simulink model "Global_control_with_arbitraty_rate_of_convergence"  (R2021a)
settings: Solver=FixedStepDiscrete  StartTime=0.0  StopTime=12  FixedStep=1.0E-5  RelTol=1e-3
undefined symbols (not defined in the file): DiscIntNeverNeededParam, sigbuilder_block
libraries: simulink x4
(part 1 of 2)
settings Model: Creator=Mehra  LastModifiedBy=Mehra

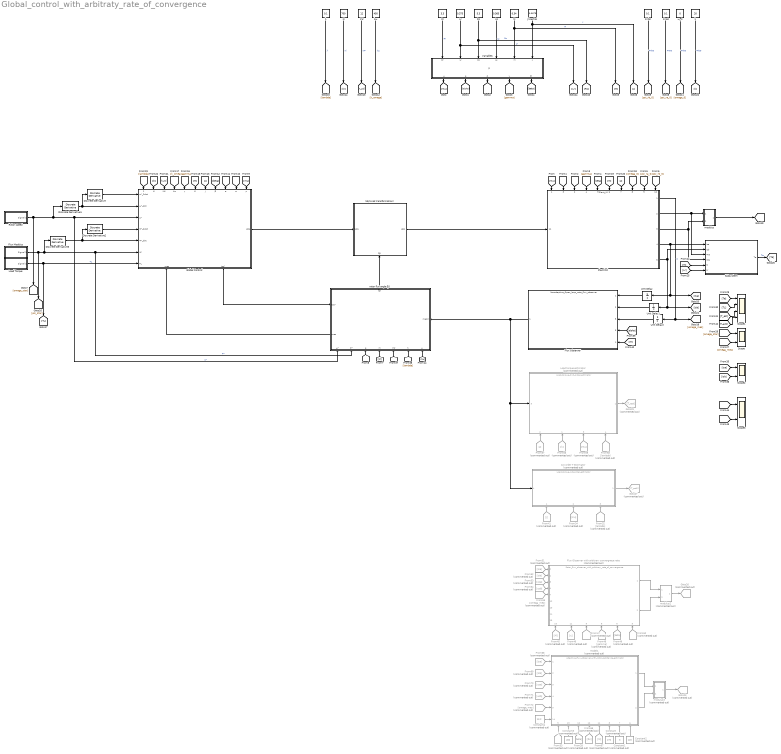
== system Global_control_with_arbitraty_rate_of_convergence ==
  note: β
  (dq to ab transformation) : Subsystem
      settings: PortSchema="{\"entries\":[{\"content\":{\"sides\":[{\"content\":{\"connectorIds\":[\"In1\"]},\"type\":\"ConnectorPlacement.EquallySpacedRectSide\",\"uuid\":\"fcc9e9c0-f3ff-45b3-b4d9-89988d9b9a34\"},{\"content\":{\"connectorIds\":[\"Out1\"],\"side\":\"RIGHT\"},\"type\":\"ConnectorPlacement.EquallySpacedRectSide\",\"uuid\":\"b8117d1c-eda8-48ca-a376-b80f3451eb1b\"},{\"content\":{\"connectorIds\":[],\"side\":\"TOP\"},\"type\":\"ConnectorPlacement.EquallySpacedRectSide\",\"uuid\":\"632a2e27-4ebf-4489-a7a1-4102ed33f7de\"},{\"content\":{\"connectorIds\":[\"In2\"],\"side\":\"BOTTOM\"},\"type\":\"ConnectorPlacement.EquallySpacedRectSide\",\"uuid\":\"b1ed2b98-7899-49a7-98d1-ff7a05505f88\"}]},\"type\":\"ConnectorPlacement.EquallySpacedConnector\",\"uuid\":\"0e689d41-d128-44ad-a484-465e7f7df4f8\"}],\"packageUris\":[\"http://schema.mathworks.com/mf0/Connector/R2020b\"],\"version\":\"1.0\"}"
  1st order T estimator : ModelReference  Commented=on  ModelNameDialog=Load_torque_1st_order_estimator.slx  SimulationMode=Normal  ModelReferenceVersion=1.13
      settings: PortSchema="{\"entries\":[{\"content\":{\"sides\":[{\"content\":{\"connectorIds\":[\"In4\"]},\"type\":\"ConnectorPlacement.EquallySpacedRectSide\",\"uuid\":\"cec251cb-6b4e-4904-a832-c5acce82a070\"},{\"content\":{\"connectorIds\":[\"Out1\"],\"side\":\"RIGHT\"},\"type\":\"ConnectorPlacement.EquallySpacedRectSide\",\"uuid\":\"735376b5-2ddd-4bd3-962c-0ec3161c2740\"},{\"content\":{\"connectorIds\":[],\"side\":\"TOP\"},\"type\":\"ConnectorPlacement.EquallySpacedRectSide\",\"uuid\":\"64a3f3a5-dee8-4d60-ac03-c9c941997ec4\"},{\"content\":{\"connectorIds\":[\"In1\",\"In2\",\"In3\"],\"side\":\"BOTTOM\"},\"type\":\"ConnectorPlacement.EquallySpacedRectSide\",\"uuid\":\"a9b1d046-d6bc-45e1-a3f0-76ce350da922\"}]},\"type\":\"ConnectorPlacement.EquallySpacedConnector\",\"uuid\":\"7512dbd3-06b9-47bd-8f2d-91bb52696950\"}],\"packageUris\":[\"http://schema.mathworks.com/mf0/Connector/R2020b\"],\"version\":\"1.0\"}"
  Constant : Constant  Commented=on  Value=270
  Constant1 : Constant  Commented=on  Value=3
  Constant2 : Constant  Commented=on  Value=120
  Constant3 : Constant  Commented=on  Value=450
  Constant4 : Constant  Commented=on  Value=13.2
  Discrete Derivative{,1..3} (4 alike) : simulink/Discrete/Discrete Derivative  gainval=1.0  ICPrevScaledInput=0.0  OutMin=[]  OutMax=[]  OutDataType=fixdt(1, 16)  OutScaling=2^-10  DoSatur=off
  Flux Modulus : Subsystem  Tag=STV Subsys  LoadFcn=sigbuilder_block('load');  StartFcn=sigbuilder_block('start');  StopFcn=sigbuilder_block('stop');  ClipboardFcn=sigbuilder_block('clipboard');  mask(Sigbuilder block){tuvar=[0:10]}
      mask help: Simulink:masks:SigbuilderBlock_MD
      mask init:
      | if ~strcmp(get_param(bdroot(gcbh),'SimulationStatus'),'stopped') tuvar = sigbuilder_block('maskInit'); end
      settings: CopyFcn=sigbuilder_block('copy');  DeleteFcn=sigbuilder_block('delete');  ModelCloseFcn=sigbuilder_block('modelClose');  PreSaveFcn=sigbuilder_block('preSave');  PauseFcn=sigbuilder_block('pause');  ContinueFcn=sigbuilder_block('continue');  NameChangeFcn=sigbuilder_block('namechange');  OpenFcn=sigbuilder_block('open',[433.8 177.6 550.8 400.2 ]);  CloseFcn=sigbuilder_block('close');
      mask Display: plot(0, 0, 100, 100,[2, 2, 32, 32, 2], [68, 8, 8, 68, 68],[32, 2], [38, 38], [32, 19, 2],[53, 60, 44], [32, 17, 17, 2],[16, 16, 31, 31]);txt = getActiveGroup(gcbh);text(2, 100, txt,'verticalAlignment', 'top');
  Flux Observer : ModelReference  ModelNameDialog=Nonadaptive_Open_loop_rotor_flux_observer  SimulationMode=Normal  ModelReferenceVersion=1.31
      settings: PortSchema="{\"entries\":[{\"content\":{\"sides\":[{\"content\":{\"connectorIds\":[\"In1\",\"In2\",\"In5\",\"In3\",\"In4\"]},\"type\":\"ConnectorPlacement.EquallySpacedRectSide\",\"uuid\":\"57c66cae-f60c-4fa2-8fd5-f5b68222e0bb\"},{\"content\":{\"connectorIds\":[\"Out1\"],\"side\":\"RIGHT\"},\"type\":\"ConnectorPlacement.EquallySpacedRectSide\",\"uuid\":\"591ff962-71a1-4adf-845c-7b897bc73935\"},{\"content\":{\"connectorIds\":[],\"side\":\"TOP\"},\"type\":\"ConnectorPlacement.EquallySpacedRectSide\",\"uuid\":\"d0e2f489-3eb5-488c-a0b4-9296b4be860b\"}]},\"type\":\"ConnectorPlacement.EquallySpacedConnector\",\"uuid\":\"15b17a83-f5fe-4267-a8df-d0f0282de86a\"}],\"packageUris\":[\"http://schema.mathworks.com/mf0/Connector/R2020b\"],\"version\":\"1.0\"}"
  Flux Observer with arbitrary convergnece rate : ModelReference  Commented=on  ModelNameDialog=Rotor_flux_observer_with_arbitrary_rate_of_convergence.slx  SimulationMode=Normal  ModelReferenceVersion=1.75
      settings: PortSchema="{\"entries\":[{\"content\":{\"sides\":[{\"content\":{\"connectorIds\":[\"In2\",\"In1\",\"In3\",\"In4\",\"In7\",\"In12\",\"In13\",\"In14\",\"In15\"]},\"type\":\"ConnectorPlacement.EquallySpacedRectSide\",\"uuid\":\"6eb1a4d5-70fa-40da-a343-d29d4ad88b11\"},{\"content\":{\"connectorIds\":[\"Out1\",\"Out2\"],\"side\":\"RIGHT\"},\"type\":\"ConnectorPlacement.EquallySpacedRectSide\",\"uuid\":\"14a59e0e-3c8f-4c9a-8db3-879e529e9be9\"},{\"content\":{\"connectorIds\":[],\"side\":\"TOP\"},\"type\":\"ConnectorPlacement.EquallySpacedRectSide\",\"uuid\":\"9bfe5fe1-910a-46f9-bc39-26e04b490667\"},{\"content\":{\"connectorIds\":[\"In10\",\"In11\",\"In9\",\"In8\",\"In6\",\"In5\"],\"side\":\"BOTTOM\"},\"type\":\"ConnectorPlacement.EquallySpacedRectSide\",\"uuid\":\"4a64a750-a430-42a9-a809-f353a68eb280\"}]},\"type\":\"ConnectorPlacement.EquallySpacedConnector\",\"uuid\":\"a7353ac2-2c9f-49b4-9477-a017cd4fcd54\"}],\"packageUris\":[\"http://schema.mathworks.com/mf0/Connector/R2020b\"],\"version\":\"1.0\"}"
  From28 : From  Commented=on  GotoTag=beta
  From32 : From  Commented=on  GotoTag=lambda
  From33 : From  Commented=on  GotoTag=sigma
  From34 : From  Commented=on  GotoTag=mu
  From41 : From  Commented=on  GotoTag=J
  From45 : From  Commented=on  GotoTag=M
  From46 : From  Commented=on  GotoTag=c
  From47 : From  Commented=on  GotoTag=sigma
  From48 : From  Commented=on  GotoTag=gamma
  From49 : From  Commented=on  GotoTag=beta
  From50 : From  Commented=on  GotoTag=alpha
  From51 : From  Commented=on  GotoTag=Isa
  From52 : From  Commented=on  GotoTag=Isb
  From53 : From  Commented=on  GotoTag=usa
  From54 : From  Commented=on  GotoTag=usb
  From55 : From  Commented=on  GotoTag=omega_mes
  From56 : From  Commented=on  GotoTag=k
  From57 : From  Commented=on  GotoTag=J
  From58 : From  Commented=on  GotoTag=lambda
  From59 : From  Commented=on  GotoTag=mu
  From66 : From  Commented=on  GotoTag=Rs
  From67 : From  Commented=on  GotoTag=M
  From68 : From  Commented=on  GotoTag=Isa
  From69 : From  Commented=on  GotoTag=Isb
  From70 : From  Commented=on  GotoTag=usa
  From71 : From  Commented=on  GotoTag=usb
  From72 : From  Commented=on  GotoTag=omega_mes
  Global Control : Subsystem
      settings: PortSchema="{\"entries\":[{\"content\":{\"sides\":[{\"content\":{\"connectorIds\":[\"In1\",\"In2\",\"In3\",\"In4\",\"In5\",\"In6\",\"In7\"]},\"type\":\"ConnectorPlacement.EquallySpacedRectSide\",\"uuid\":\"d7ac22ed-73dc-4923-8a02-de2b77bc4b56\"},{\"content\":{\"connectorIds\":[\"Out1\"],\"side\":\"RIGHT\"},\"type\":\"ConnectorPlacement.EquallySpacedRectSide\",\"uuid\":\"0ed82d2d-ac01-4440-b414-7b739c3193d9\"},{\"content\":{\"connectorIds\":[\"In8\",\"In9\",\"In10\",\"In11\",\"In12\",\"In13\",\"In14\",\"In15\",\"In16\",\"In17\",\"In18\"],\"side\":\"TOP\"},\"type\":\"ConnectorPlacement.EquallySpacedRectSide\",\"uuid\":\"be3374af-951c-49b1-9762-82694f1e2186\"},{\"content\":{\"connectorIds\":[\"In19\",\"Out2\"],\"side\":\"BOTTOM\"},\"type\":\"ConnectorPlacement.EquallySpacedRectSide\",\"uuid\":\"0e0cdf13-df45-4d83-96ab-036d988b30e8\"}]},\"type\":\"ConnectorPlacement.EquallySpacedConnector\",\"uuid\":\"01640f11-0e41-43e3-9a6d-1e07964cb7e3\"}],\"packageUris\":[\"http://schema.mathworks.com/mf0/Connector/R2020b\"],\"version\":\"1.0\"}"
  Goto23 : Goto  Commented=on  GotoTag=psi_est2
  Goto26 : Goto  Commented=on  GotoTag=psi_est2
  Goto27 : Goto  Commented=on  GotoTag=T_est2
  Goto29 : Goto  Commented=on  GotoTag=T_est
  J(inertia) : Constant  Value=0.0075
  Ki : Constant  Value=700
  KΨ : Constant  Value=12
  Load Torque : Subsystem  Tag=STV Subsys  LoadFcn=sigbuilder_block('load');  StartFcn=sigbuilder_block('start');  StopFcn=sigbuilder_block('stop');  ClipboardFcn=sigbuilder_block('clipboard');  mask(Sigbuilder block){tuvar=[0:10]}
      mask help: Simulink:masks:SigbuilderBlock_MD
      mask init:
      | if ~strcmp(get_param(bdroot(gcbh),'SimulationStatus'),'stopped') tuvar = sigbuilder_block('maskInit'); end
      settings: CopyFcn=sigbuilder_block('copy');  DeleteFcn=sigbuilder_block('delete');  ModelCloseFcn=sigbuilder_block('modelClose');  PreSaveFcn=sigbuilder_block('preSave');  PauseFcn=sigbuilder_block('pause');  ContinueFcn=sigbuilder_block('continue');  NameChangeFcn=sigbuilder_block('namechange');  OpenFcn=sigbuilder_block('open',[418.2 149.4 550.8 400.2 ]);  CloseFcn=sigbuilder_block('close');
      mask Display: plot(0, 0, 100, 100,[2, 2, 32, 32, 2], [68, 8, 8, 68, 68],[32, 2], [38, 38], [32, 19, 2],[53, 60, 44], [32, 17, 17, 2],[16, 16, 31, 31]);txt = getActiveGroup(gcbh);text(2, 100, txt,'verticalAlignment', 'top');
  Load torque estimator : ModelReference  Commented=on  ModelNameDialog=Load_torque_2nd_order_estimator  SimulationMode=Normal  ModelReferenceVersion=1.28
      settings: PortSchema="{\"entries\":[{\"content\":{\"sides\":[{\"content\":{\"connectorIds\":[\"In5\"]},\"type\":\"ConnectorPlacement.EquallySpacedRectSide\",\"uuid\":\"6c630a82-6d29-475e-ba8f-daf1e6858c20\"},{\"content\":{\"connectorIds\":[\"Out1\"],\"side\":\"RIGHT\"},\"type\":\"ConnectorPlacement.EquallySpacedRectSide\",\"uuid\":\"ccfb3e1f-a267-4346-837b-0235b5167929\"},{\"content\":{\"connectorIds\":[],\"side\":\"TOP\"},\"type\":\"ConnectorPlacement.EquallySpacedRectSide\",\"uuid\":\"2167c938-58ec-47d6-a980-0c72b06e2cda\"},{\"content\":{\"connectorIds\":[\"In2\",\"In1\",\"In3\",\"In4\"],\"side\":\"BOTTOM\"},\"type\":\"ConnectorPlacement.EquallySpacedRectSide\",\"uuid\":\"b11c489e-5397-4870-bc2b-0329756c8e12\"}]},\"type\":\"ConnectorPlacement.EquallySpacedConnector\",\"uuid\":\"6322234a-0e23-4641-96ea-e8bbbfd716bb\"}],\"packageUris\":[\"http://schema.mathworks.com/mf0/Connector/R2020b\"],\"version\":\"1.0\"}"
  Lr : Constant  Value=0.375
  Ls : Constant  Value=0.365
  M : Constant  Value=0.34
  Model1 : ModelReference  Commented=on  ModelNameDialog=Adaptive_flux_observer_with_rotor_resistance_estimator.slx  SimulationMode=Normal  ModelReferenceVersion=1.192
      settings: PortSchema="{\"entries\":[{\"content\":{\"sides\":[{\"content\":{\"connectorIds\":[\"In1\",\"In2\",\"In3\",\"In4\",\"In5\",\"In14\"]},\"type\":\"ConnectorPlacement.EquallySpacedRectSide\",\"uuid\":\"0dfbc06b-2b07-4b1e-b8bc-3256d137db57\"},{\"content\":{\"connectorIds\":[\"Out1\",\"Out2\"],\"side\":\"RIGHT\"},\"type\":\"ConnectorPlacement.EquallySpacedRectSide\",\"uuid\":\"bd842826-8417-4de1-9520-786241a65cac\"},{\"content\":{\"connectorIds\":[],\"side\":\"TOP\"},\"type\":\"ConnectorPlacement.EquallySpacedRectSide\",\"uuid\":\"d4d18e1c-2da3-42ce-bbd2-432513d498b9\"},{\"content\":{\"connectorIds\":[\"In9\",\"In13\",\"In10\",\"In12\",\"In11\",\"In8\",\"In7\",\"In6\"],\"side\":\"BOTTOM\"},\"type\":\"ConnectorPlacement.EquallySpacedRectSide\",\"uuid\":\"5bcd1c2a-69a8-47f4-8b62-1a55c0f1a24c\"}]},\"type\":\"ConnectorPlacement.EquallySpacedConnector\",\"uuid\":\"5c441b24-ee71-4b77-81dd-97c2eaa661e7\"}],\"packageUris\":[\"http://schema.mathworks.com/mf0/Connector/R2020b\"],\"version\":\"1.0\"}"
  Plant(IM) : ModelReference  ModelNameDialog=Plant_IM  SimulationMode=Normal  ModelReferenceVersion=1.73
      settings: PortSchema="{\"entries\":[{\"content\":{\"sides\":[{\"content\":{\"connectorIds\":[\"In11\"]},\"type\":\"ConnectorPlacement.EquallySpacedRectSide\",\"uuid\":\"c1ced4ac-9292-447b-a16b-48862d3db151\"},{\"content\":{\"connectorIds\":[\"Out1\",\"Out2\",\"Out3\",\"Out4\",\"Out5\"],\"side\":\"RIGHT\"},\"type\":\"ConnectorPlacement.EquallySpacedRectSide\",\"uuid\":\"13a72579-fb39-4c86-8f38-f8272c138e74\"},{\"content\":{\"connectorIds\":[\"In1\",\"In3\",\"In2\",\"In4\",\"In5\",\"In6\",\"In7\",\"In8\",\"In9\",\"In10\"],\"side\":\"TOP\"},\"type\":\"ConnectorPlacement.EquallySpacedRectSide\",\"uuid\":\"7112169d-3c72-435f-89ee-d1fe7807fab2\"}]},\"type\":\"ConnectorPlacement.EquallySpacedConnector\",\"uuid\":\"c43df563-9598-43b0-9064-e7550f78106e\"}],\"packageUris\":[\"http://schema.mathworks.com/mf0/Connector/R2020b\"],\"version\":\"1.0\"}"
  Rotor speed : Subsystem  Tag=STV Subsys  LoadFcn=sigbuilder_block('load');  StartFcn=sigbuilder_block('start');  StopFcn=sigbuilder_block('stop');  ClipboardFcn=sigbuilder_block('clipboard');  mask(Sigbuilder block){tuvar=[0:10]}
      mask help: Simulink:masks:SigbuilderBlock_MD
      mask init:
      | if ~strcmp(get_param(bdroot(gcbh),'SimulationStatus'),'stopped') tuvar = sigbuilder_block('maskInit'); end
      settings: CopyFcn=sigbuilder_block('copy');  DeleteFcn=sigbuilder_block('delete');  ModelCloseFcn=sigbuilder_block('modelClose');  PreSaveFcn=sigbuilder_block('preSave');  PauseFcn=sigbuilder_block('pause');  ContinueFcn=sigbuilder_block('continue');  NameChangeFcn=sigbuilder_block('namechange');  OpenFcn=sigbuilder_block('open',[418.2 149.4 550.8 400.2 ]);  CloseFcn=sigbuilder_block('close');
      mask Display: plot(0, 0, 100, 100,[2, 2, 32, 32, 2], [68, 8, 8, 68, 68],[32, 2], [38, 38], [32, 19, 2],[53, 60, 44], [32, 17, 17, 2],[16, 16, 31, 31]);txt = getActiveGroup(gcbh);text(2, 100, txt,'verticalAlignment', 'top');
  Rr : Constant  Value=3.3
  Rs : Constant  Value=5.3
  Scope : Scope  NumInputPorts=2
  Scope1 : Scope  NumInputPorts=4
  Scope2 : Scope  NumInputPorts=2
  Scope3 : Scope  NumInputPorts=2
  Subsystem : Subsystem
  Unit Delay : UnitDelay  SampleTime=-1  HasFrameUpgradeWarning=on
  Unit Delay1 : UnitDelay  SampleTime=-1  HasFrameUpgradeWarning=on
  Unit Delay2 : UnitDelay  SampleTime=-1  HasFrameUpgradeWarning=on
  Variables : Subsystem
  k : Constant  Value=20
  kω : Constant  Value=450
  modulus : Subsystem
  modulus2 : Subsystem  Commented=on
  modulus3 : Subsystem  Commented=on
  rotor flux angle ξ0 : Subsystem
      settings: PortSchema="{\"entries\":[{\"content\":{\"sides\":[{\"content\":{\"connectorIds\":[\"In1\",\"Out2\"]},\"type\":\"ConnectorPlacement.EquallySpacedRectSide\",\"uuid\":\"954ddc6c-32ec-4fca-997a-51b3ced09e6e\"},{\"content\":{\"connectorIds\":[\"In9\"],\"side\":\"RIGHT\"},\"type\":\"ConnectorPlacement.EquallySpacedRectSide\",\"uuid\":\"d23f0106-fd66-41c5-9167-f0bfa2e5f0d7\"},{\"content\":{\"connectorIds\":[\"Out1\"],\"side\":\"TOP\"},\"type\":\"ConnectorPlacement.EquallySpacedRectSide\",\"uuid\":\"ec2ab734-74ce-4c08-89a8-e0d0cab377a3\"},{\"content\":{\"connectorIds\":[\"In2\",\"In3\",\"In4\",\"In5\",\"In6\",\"In7\",\"In8\"],\"side\":\"BOTTOM\"},\"type\":\"ConnectorPlacement.EquallySpacedRectSide\",\"uuid\":\"e8fbabf1-c1e7-4b41-8038-4f25f2d2c141\"}]},\"type\":\"ConnectorPlacement.EquallySpacedConnector\",\"uuid\":\"2eb72d65-4150-4441-ba17-035a64db8a78\"}],\"packageUris\":[\"http://schema.mathworks.com/mf0/Connector/R2020b\"],\"version\":\"1.0\"}"
  Ψra0 : Constant  Value=0.1
  Ψrb0 : Constant  Value=0.1
  λ : Constant  Value=0.1
  ω_0 : Constant  Value=0
  wires:
  Variables/5(β) -> [beta]
  Rr/1 -> Variables/1(Rr)  "Rr"
  Ψra0/1 -> [psi_ra_0]  "Ψra0"
  Variables/2(α) -> [alpha]
  J(inertia)/1 -> [J], Variables/6(J)  "J"
  Ls/1 -> Variables/4(Ls)  "Ls"
  ω_0/1 -> [omega_0]  "Ψrb0"
  [psi_rb_0] -> Plant(IM)/10
  Lr/1 -> [Lr], Variables/2(Lr)  "Lr"
  [psi_ra_0] -> Plant(IM)/9
  Variables/3(σ) -> [sigma]
  Rs/1 -> [Rs], Variables/3(Rs)  "Rs"
  Variables/4(γ) -> [gamma]
  Variables/1(µ) -> [mu]
  Ψrb0/1 -> [psi_rb_0]  "Ψrb0"
  M/1 -> [M], Variables/5(M)  "M"
  Ki/1 -> [ki]  "Ki"
  kω/1 -> [k_omega]  "kω"
  KΨ/1 -> [K_psi]  "KΨ"
  λ/1 -> [lambda]  "λ"
  [M] -> rotor flux angle ξ0/5(M)
  [alpha] -> rotor flux angle ξ0/4(α)
  Plant(IM)/1 -> [omega_mes], Unit Delay2/1  "ω"
  Plant(IM)/3 -> modulus/2(In2), Subsystem/4(Ψrb)
  Plant(IM)/4 -> [Isa], Unit Delay/1, Subsystem/1(Isa)
  Plant(IM)/5 -> Subsystem/2(Isb), Unit Delay1/1, [Isb]
  Rotor speed/1(Signal 1) -> Global Control/3(ω*), rotor flux angle ξ0/2(ω*), Discrete Derivative1/1, [omega_star]  "ω*"
  Flux Modulus/1(Signal 1) -> Discrete Derivative3/1, Global Control/6(Ψ*), rotor flux angle ξ0/3(Ψ*), [psi_star]  "Ψ*"
  Load Torque/1(Signal 1) -> Global Control/7(TL), [TL]  "TL"
  Discrete Derivative3/1 -> Discrete Derivative2/1, Global Control/5(Ψ*_dot)
  Discrete Derivative2/1 -> Global Control/4(Ψ*_2dot)
  Discrete Derivative/1 -> Global Control/1(ω*_2dot)
  Discrete Derivative1/1 -> Discrete Derivative/1, Global Control/2(ω*_dot)
  [mu] -> Global Control/18(µ)
  [alpha] -> Global Control/17(α)
  [sigma] -> Global Control/16(σ)
  [beta] -> Global Control/15(β)
  [J] -> Global Control/14(J)
  [M] -> Global Control/13(M)
  [gamma] -> Global Control/12(γ)
  [k_omega] -> Global Control/11(Kω)
  [K_psi] -> Global Control/10(KΨ)
  [ki] -> Global Control/9(Ki)
  [lambda] -> Global Control/8(λ)
  [omega_star] -> Scope/1
  [omega_mes] -> Scope/2
  [Isa] -> Scope2/1
  [Isb] -> Scope2/2
  modulus/1(Out1) -> [psi_mes]
  [alpha] -> Flux Observer/3
  [M] -> Flux Observer/4
  From45/1 -> Flux Observer with arbitrary convergnece rate/10
  From46/1 -> Flux Observer with arbitrary convergnece rate/11
  From47/1 -> Flux Observer with arbitrary convergnece rate/9
  From48/1 -> Flux Observer with arbitrary convergnece rate/8
  From49/1 -> Flux Observer with arbitrary convergnece rate/6
  From50/1 -> Flux Observer with arbitrary convergnece rate/5
  From51/1 -> Flux Observer with arbitrary convergnece rate/2
  From52/1 -> Flux Observer with arbitrary convergnece rate/1
  From53/1 -> Flux Observer with arbitrary convergnece rate/3
  From54/1 -> Flux Observer with arbitrary convergnece rate/4
  From55/1 -> Flux Observer with arbitrary convergnece rate/7
  modulus2/1(Out1) -> Goto26/1
  Flux Observer with arbitrary convergnece rate/1 -> modulus2/1(Ψra_est)
  Flux Observer with arbitrary convergnece rate/2 -> modulus2/2(Ψrb_est)
  From58/1 -> Load torque estimator/4
  From59/1 -> Load torque estimator/3
  Load torque estimator/1 -> Goto29/1
  From28/1 -> Model1/10
  From33/1 -> Model1/9
  From66/1 -> Model1/12
  From67/1 -> Model1/11
  Constant/1 -> Model1/8
  Constant1/1 -> Model1/7
  Constant2/1 -> Model1/6
  Constant3/1 -> Model1/13
  From68/1 -> Model1/1
  From69/1 -> Model1/2
  From70/1 -> Model1/3
  From71/1 -> Model1/4
  From72/1 -> Model1/5
  modulus3/1(Out1) -> Goto23/1
  Model1/1 -> modulus3/1(Ψra_est)
  Model1/2 -> modulus3/2(Ψrb_est)
  Constant4/1 -> Model1/14
  Plant(IM)/2 -> Subsystem/3(Ψra), modulus/1(Ψra)
  rotor flux angle ξ0/1(ξ0) -> (dq to ab transformation)/2(ξ0)
  [mu] -> rotor flux angle ξ0/8(µ)
  [K_psi] -> rotor flux angle ξ0/6(KΨ)
  [lambda] -> rotor flux angle ξ0/7(λ)
  Global Control/2(Isq*) -> rotor flux angle ξ0/1(Isq*)
  [M] -> Subsystem/5(M)
  rotor flux angle ξ0/2(mes) -> Global Control/19(mes)
  [Lr] -> Subsystem/6(Lr)
  Subsystem/1(Te) -> [Te]  "Te"
  [psi_star] -> Scope3/1
  [psi_mes] -> Scope3/2
  [TL] -> Scope1/2
  [Te] -> Scope1/1
  Unit Delay1/1 -> Flux Observer/2
  Flux Observer/1 -> 1st order T estimator/4, Load torque estimator/5, rotor flux angle ξ0/9(mesin)
  Global Control/1(Udq) -> (dq to ab transformation)/1(Udq)
  (dq to ab transformation)/1(Uab) -> Plant(IM)/11
  [M] -> Plant(IM)/6
  [omega_0] -> Plant(IM)/8
  [J] -> Plant(IM)/7
  [beta] -> Plant(IM)/5
  [gamma] -> Plant(IM)/4
  [alpha] -> Plant(IM)/2
  [sigma] -> Plant(IM)/3
  [mu] -> Plant(IM)/1
  From57/1 -> Load torque estimator/2
  From56/1 -> Load torque estimator/1
  k/1 -> [k]  "Ψrb0"
  [T_est] -> Scope1/3
  Unit Delay/1 -> Flux Observer/1
  Unit Delay2/1 -> Flux Observer/5
  From32/1 -> 1st order T estimator/3
  From34/1 -> 1st order T estimator/2
  From41/1 -> 1st order T estimator/1
  1st order T estimator/1 -> Goto27/1
  [T_est2] -> Scope1/4

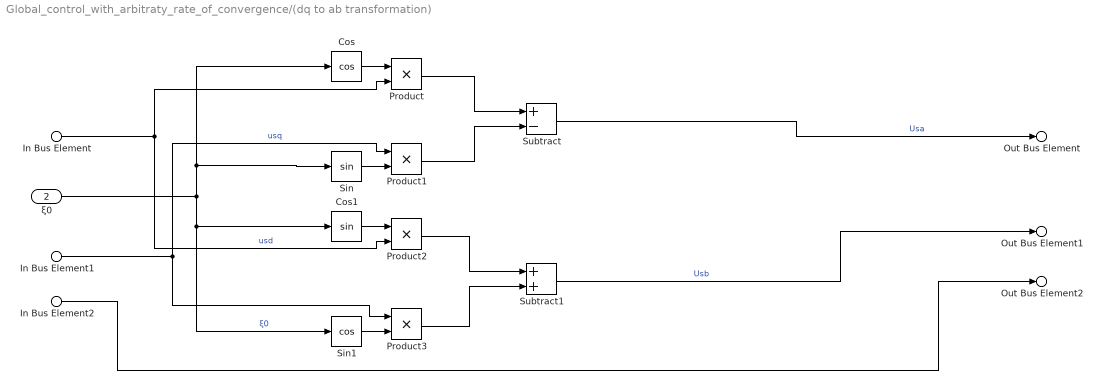
== system Global_control_with_arbitraty_rate_of_convergence/(dq to ab transformation) ==
  In Bus Element : Inport  PortName=Udq  Element=usd
  In Bus Element1 : Inport  PortName=Udq  Element=usq
  In Bus Element2 : Inport  PortName=Udq  Element=TL
  ξ0 : Inport  Port=2
  Cos : Trigonometry  Operator=cos
  Cos1 : Trigonometry
  Product{,1..3} (4 alike) : Product
  Sin : Trigonometry
  Sin1 : Trigonometry  Operator=cos
  Subtract : Sum  Inputs=+-
  Subtract1 : Sum
  Out Bus Element : Outport  PortName=Uab  Element=Usa
  Out Bus Element1 : Outport  PortName=Uab  Element=Usb
  Out Bus Element2 : Outport  PortName=Uab  Element=TL
  wires:
  Subtract1/1 -> Out Bus Element1/1  "Usb"
  Subtract/1 -> Out Bus Element/1  "Usa"
  ξ0/1 -> Sin1/1, Cos1/1, Sin/1, Cos/1  "ξ0"
  Cos/1 -> Product/1
  Sin/1 -> Product1/2
  Cos1/1 -> Product2/1
  Sin1/1 -> Product3/2
  In Bus Element/1 -> Product2/2, Product/2  "usd"
  In Bus Element1/1 -> Product3/1, Product1/1  "usq"
  Product/1 -> Subtract/1
  Product1/1 -> Subtract/2
  Product2/1 -> Subtract1/1
  Product3/1 -> Subtract1/2
  In Bus Element2/1 -> Out Bus Element2/1

== system Global_control_with_arbitraty_rate_of_convergence/Flux Modulus ==
  Demux : Demux  Tag=STV Demux  Outputs=1
      settings: DisplayOption=none
  FromWs : FromWorkspace  Tag=STV FromWs  VariableName=tuvar
      SigBuilderData=|
      | common.afterFinalStr = 'Extrapolate'
      | common.sampleTime = 0
      | dataSet.timeRange = [0 10]
      | dataSet.name = 'Group 1'
      | sbobj.Groups.Name = 'Group 1'
      | sbobj.Groups.Signals.Name = 'Signal 1'
      | sbobj.Groups.Signals.XData = [0 0.32 1.5 1.8 10]
      | sbobj.Groups.Signals.YData = [0.001 1.16 1.16 0.5 0.5]
  Signal 1 : Outport  Tag=STV Outport
  wires:
  Demux/1 -> Signal 1/1
  FromWs/1 -> Demux/1

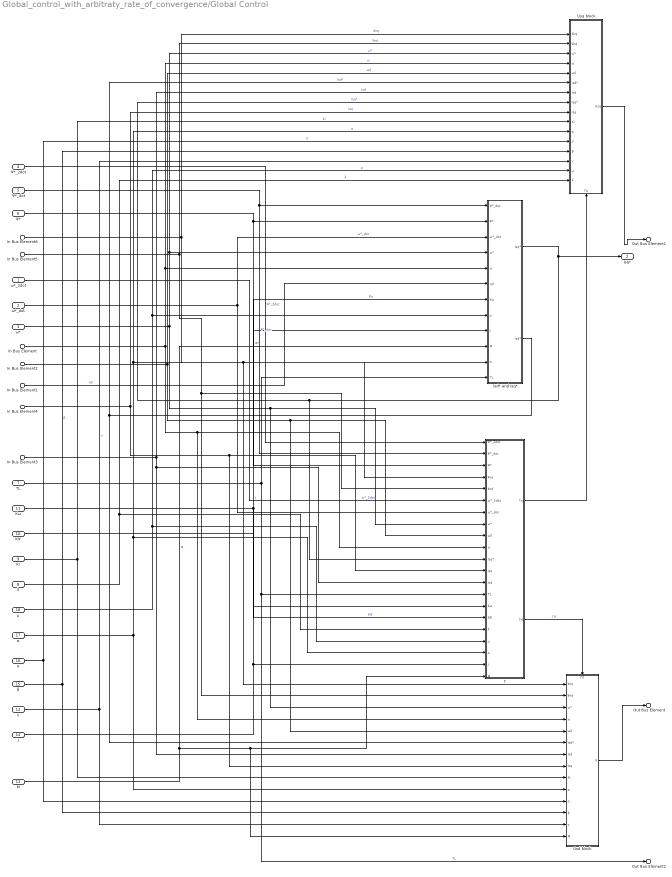
== system Global_control_with_arbitraty_rate_of_convergence/Global Control ==
  ω*_2dot : Inport
  ω*_dot : Inport  Port=2
  ω* : Inport  Port=3
  Ψ*_2dot : Inport  Port=4
  Ψ*_dot : Inport  Port=5
  Ψ* : Inport  Port=6
  TL : Inport  Port=7
  λ : Inport  Port=8
  Ki : Inport  Port=9
  KΨ : Inport  Port=10
  Kω : Inport  Port=11
  γ : Inport  Port=12
  M : Inport  Port=13
  J : Inport  Port=14
  β : Inport  Port=15
  σ : Inport  Port=16
  α : Inport  Port=17
  µ : Inport  Port=18
  In Bus Element : Inport  Port=19  PortName=mes  Element=ω
  In Bus Element1 : Inport  Port=19  PortName=mes  Element=ηd
  In Bus Element2 : Inport  Port=19  PortName=mes  Element=ω0
  In Bus Element3 : Inport  Port=19  PortName=mes  Element=Isd
  In Bus Element4 : Inport  Port=19  PortName=mes  Element=Isq
  In Bus Element5 : Inport  Port=19  PortName=mes  Element=Ψrd
  In Bus Element6 : Inport  Port=19  PortName=mes  Element=Ψrq
  Isd* and Isq* : Subsystem
  Usd block : Subsystem
      settings: PortSchema="{\"entries\":[{\"content\":{\"sides\":[{\"content\":{\"connectorIds\":[\"In1\",\"In2\",\"In3\",\"In4\",\"In5\",\"In6\",\"In7\",\"In8\",\"In9\",\"In10\",\"In11\",\"In12\",\"In13\",\"In14\"]},\"type\":\"ConnectorPlacement.EquallySpacedRectSide\",\"uuid\":\"0b3b8e54-774f-4e59-b7ae-fc3f76f7169f\"},{\"content\":{\"connectorIds\":[\"Out1\"],\"side\":\"RIGHT\"},\"type\":\"ConnectorPlacement.EquallySpacedRectSide\",\"uuid\":\"160f327c-323c-4922-a7f8-789847ab983f\"},{\"content\":{\"connectorIds\":[\"In15\"],\"side\":\"TOP\"},\"type\":\"ConnectorPlacement.EquallySpacedRectSide\",\"uuid\":\"f6ec24e2-9a41-47bb-ba15-6aba8409f45e\"}]},\"type\":\"ConnectorPlacement.EquallySpacedConnector\",\"uuid\":\"52a2cf74-17c5-48e5-8a86-53458a7f2c84\"}],\"packageUris\":[\"http://schema.mathworks.com/mf0/Connector/R2020b\"],\"version\":\"1.0\"}"
  Usq block : Subsystem
      settings: PortSchema="{\"entries\":[{\"content\":{\"sides\":[{\"content\":{\"connectorIds\":[\"In1\",\"In2\",\"In3\",\"In4\",\"In5\",\"In6\",\"In7\",\"In8\",\"In9\",\"In10\",\"In11\",\"In12\",\"In13\",\"In14\",\"In15\",\"In16\"]},\"type\":\"ConnectorPlacement.EquallySpacedRectSide\",\"uuid\":\"e0829cb0-14ba-4968-8b37-82965b41b0aa\"},{\"content\":{\"connectorIds\":[\"Out1\"],\"side\":\"RIGHT\"},\"type\":\"ConnectorPlacement.EquallySpacedRectSide\",\"uuid\":\"1d4d172a-7610-496b-b8fe-18e12381e6b4\"},{\"content\":{\"connectorIds\":[],\"side\":\"TOP\"},\"type\":\"ConnectorPlacement.EquallySpacedRectSide\",\"uuid\":\"0fc98001-c07f-432d-975f-c7605f9f4273\"},{\"content\":{\"connectorIds\":[\"In17\"],\"side\":\"BOTTOM\"},\"type\":\"ConnectorPlacement.EquallySpacedRectSide\",\"uuid\":\"89865e84-6121-4a9b-9592-d6a2eae0e50b\"}]},\"type\":\"ConnectorPlacement.EquallySpacedConnector\",\"uuid\":\"d7e7f672-cce9-4dd7-86e0-c30144b95288\"}],\"packageUris\":[\"http://schema.mathworks.com/mf0/Connector/R2020b\"],\"version\":\"1.0\"}"
  Γ : Subsystem
  Out Bus Element : Outport  PortName=Udq  Element=usd
  Out Bus Element1 : Outport  PortName=Udq  Element=usq
  Out Bus Element2 : Outport  PortName=Udq  Element=TL
  Isq* : Outport  Port=2
  wires:
  Ψ*_2dot/1 -> Γ/1(Ψ*_2dot)  "Ψ*_2dot"
  Ψ*_dot/1 -> Isd* and Isq*/1(Ψ*_dot), Γ/2(Ψ*_dot)  "Ψ*_dot"
  Ψ*/1 -> Isd* and Isq*/2(Ψ*), Γ/3(Ψ*)  "Ψ*"
  In Bus Element6/1 -> Usq block/1(Ψrq), Γ/4(Ψrq), Usd block/1(Ψrq)  "Ψrq"
  In Bus Element5/1 -> Usq block/2(Ψrd), Γ/5(Ψrd), Usd block/2(Ψrd)  "Ψrd"
  ω*_2dot/1 -> Γ/6(ω*_2dot)  "ω*_2dot"
  ω*_dot/1 -> Isd* and Isq*/3(ω*_dot), Γ/7(ω*_dot)  "ω*_dot"
  ω*/1 -> Usd block/3(ω*), Γ/8(ω*), Isd* and Isq*/4(ω*), Usq block/3(ω*)  "ω*"
  In Bus Element2/1 -> Usq block/5(ω0), Usd block/5(ω0), Γ/9(ω0)  "ω0"
  In Bus Element/1 -> Usd block/4(ω), Γ/10(ω), Isd* and Isq*/5(ω), Usq block/4(ω)  "ω"
  Isd* and Isq*/1(Isq*) -> Isq*/1, Usq block/8(Isq*), Γ/11(Isq*)  "Isq*"
  In Bus Element4/1 -> Usq block/9(Isq), Γ/12(Isq), Usd block/8(Isq)  "Isq"
  In Bus Element3/1 -> Usq block/7(Isd), Γ/13(Isd), Usd block/7(Isd)  "Isd"
  TL/1 -> Isd* and Isq*/12(TL), Out Bus Element2/1, Γ/14(TL)  "TL"
  Kω/1 -> Γ/15(Kω), Isd* and Isq*/7(Kω)  "Kω"
  KΨ/1 -> Γ/16(KΨ)  "KΨ"
  λ/1 -> Γ/17(λ), Usq block/16(λ)  "λ"
  µ/1 -> Isd* and Isq*/8(µ), Usq block/15(µ), Γ/18(µ)  "µ"
  α/1 -> Γ/19(α), Usq block/11(α), Isd* and Isq*/11(α), Usd block/10(α)  "α"
  J/1 -> Γ/20(J), Isd* and Isq*/9(J)  "J"
  M/1 -> Isd* and Isq*/10(M), Γ/21(M), Usd block/14(M)  "M"
  Isd* and Isq*/2(Isd*) -> Usd block/6(Isd*), Usq block/6(Isd*)  "Isd*"
  Γ/2(Γd) -> Usd block/15(Γd)  "Γd"
  Ki/1 -> Usq block/10(Ki), Usd block/9(Ki)  "Ki"
  σ/1 -> Usq block/12(σ), Usd block/11(σ)  "σ"
  β/1 -> Usq block/13(β), Usd block/12(β)  "β"
  γ/1 -> Usq block/14(γ), Usd block/13(γ)  "γ"
  Usd block/1(U) -> Out Bus Element/1
  Γ/1(Γq) -> Usq block/17(Γq)
  Usq block/1(Usq) -> Out Bus Element1/1
  In Bus Element1/1 -> Isd* and Isq*/6(ηd)  "ηd"

== system Global_control_with_arbitraty_rate_of_convergence/Load Torque ==
  Demux : Demux  Tag=STV Demux  Outputs=1
      settings: DisplayOption=none
  FromWs : FromWorkspace  Tag=STV FromWs  VariableName=tuvar
      SigBuilderData=|
      | common.afterFinalStr = 'Extrapolate'
      | common.sampleTime = 0
      | dataSet.timeRange = [0 10]
      | dataSet.name = 'Group 1'
      | sbobj.Groups.Name = 'Group 1'
      | sbobj.Groups.Signals.Name = 'Signal 1'
      | sbobj.Groups.Signals.XData = [0 0.32 0.32 1 1 10]
      | sbobj.Groups.Signals.YData = [0 0 5.8 5.8 1.8 1.8]
  Signal 1 : Outport  Tag=STV Outport
  wires:
  Demux/1 -> Signal 1/1
  FromWs/1 -> Demux/1

== system Global_control_with_arbitraty_rate_of_convergence/Rotor speed ==
  Demux : Demux  Tag=STV Demux  Outputs=1
      settings: DisplayOption=none
  FromWs : FromWorkspace  Tag=STV FromWs  VariableName=tuvar
      SigBuilderData=|
      | common.afterFinalStr = 'Extrapolate'
      | common.sampleTime = 0
      | dataSet.timeRange = [0 10]
      | dataSet.name = 'Group 1'
      | sbobj.Groups.Name = 'Group 1'
      | sbobj.Groups.Signals.Name = 'Signal 1'
      | sbobj.Groups.Signals.XData = [0 0.32 1 1.5 2 10]
      | sbobj.Groups.Signals.YData = [0 0 100 100 200 200]
  Signal 1 : Outport  Tag=STV Outport
  wires:
  Demux/1 -> Signal 1/1
  FromWs/1 -> Demux/1

== system Global_control_with_arbitraty_rate_of_convergence/Subsystem ==
  Isa : Inport
  Isb : Inport  Port=2
  Ψra : Inport  Port=3
  Ψrb : Inport  Port=4
  M : Inport  Port=5
  Lr : Inport  Port=6
  Add : Sum  Inputs=+-
  Product : Product  Inputs=**/
  Product1 : Product
  Product2 : Product
  Te : Outport
  wires:
  Product/1 -> Te/1
  Add/1 -> Product/1
  M/1 -> Product/2
  Lr/1 -> Product/3
  Product1/1 -> Add/1
  Product2/1 -> Add/2
  Ψra/1 -> Product1/1
  Isb/1 -> Product1/2
  Ψrb/1 -> Product2/2
  Isa/1 -> Product2/1

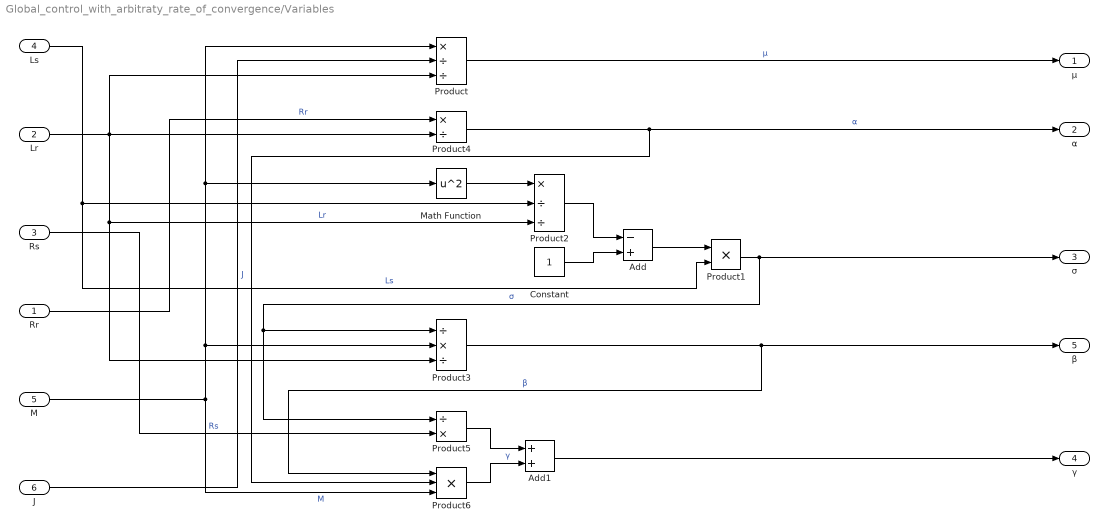
== system Global_control_with_arbitraty_rate_of_convergence/Variables ==
  Rr : Inport
  Lr : Inport  Port=2
  Rs : Inport  Port=3
  Ls : Inport  Port=4
  M : Inport  Port=5
  J : Inport  Port=6
  Add : Sum  Inputs=-+
  Add1 : Sum
  Constant : Constant
  Math Function : Math  Operator=square  SaturateOnIntegerOverflow=on
  Product : Product  Inputs=*//
  Product1 : Product
  Product2 : Product  Inputs=*//
  Product3 : Product  Inputs=/*/
  Product4 : Product  Inputs=*/
  Product5 : Product  Inputs=/*
  Product6 : Product  Inputs=3
  µ : Outport
  α : Outport  Port=2
  σ : Outport  Port=3
  γ : Outport  Port=4
  β : Outport  Port=5
  wires:
  M/1 -> Product3/2, Math Function/1, Product/1, Product6/3  "M"
  J/1 -> Product/2  "J"
  Lr/1 -> Product4/2, Product/3, Product2/3, Product3/3  "Lr"
  Product/1 -> µ/1  "µ"
  Add/1 -> Product1/1
  Ls/1 -> Product2/2, Product1/2  "Ls"
  Product1/1 -> Product3/1, Product5/1, σ/1  "σ"
  Constant/1 -> Add/2
  Product2/1 -> Add/1
  Math Function/1 -> Product2/1
  Product3/1 -> Product6/1, β/1  "β"
  Rr/1 -> Product4/1  "Rr"
  Product4/1 -> Product6/2, α/1  "α"
  Rs/1 -> Product5/2  "Rs"
  Product6/1 -> Add1/2  "γ"
  Product5/1 -> Add1/1
  Add1/1 -> γ/1

== system Global_control_with_arbitraty_rate_of_convergence/modulus ==
  Ψra : Inport
  In2 : Inport  Port=2
  Add : Sum
  Math Function : Math  Operator=square  SaturateOnIntegerOverflow=on
  Math Function1 : Math  Operator=square  SaturateOnIntegerOverflow=on
  Sqrt : Sqrt  SaturateOnIntegerOverflow=on
  Out1 : Outport
  wires:
  Add/1 -> Sqrt/1
  In2/1 -> Math Function1/1
  Ψra/1 -> Math Function/1
  Math Function1/1 -> Add/2
  Math Function/1 -> Add/1
  Sqrt/1 -> Out1/1

== system Global_control_with_arbitraty_rate_of_convergence/modulus2 ==
  Ψra_est : Inport
  Ψrb_est : Inport  Port=2
  Add : Sum
  Math Function : Math  Operator=square  SaturateOnIntegerOverflow=on
  Math Function1 : Math  Operator=square  SaturateOnIntegerOverflow=on
  Sqrt : Sqrt  SaturateOnIntegerOverflow=on
  Out1 : Outport
  wires:
  Add/1 -> Sqrt/1
  Ψrb_est/1 -> Math Function1/1
  Ψra_est/1 -> Math Function/1
  Math Function1/1 -> Add/2
  Math Function/1 -> Add/1
  Sqrt/1 -> Out1/1

== system Global_control_with_arbitraty_rate_of_convergence/modulus3 ==
  Ψra_est : Inport
  Ψrb_est : Inport  Port=2
  Add : Sum
  Math Function : Math  Operator=square  SaturateOnIntegerOverflow=on
  Math Function1 : Math  Operator=square  SaturateOnIntegerOverflow=on
  Sqrt : Sqrt  SaturateOnIntegerOverflow=on
  Out1 : Outport
  wires:
  Add/1 -> Sqrt/1
  Ψrb_est/1 -> Math Function1/1
  Ψra_est/1 -> Math Function/1
  Math Function1/1 -> Add/2
  Math Function/1 -> Add/1
  Sqrt/1 -> Out1/1

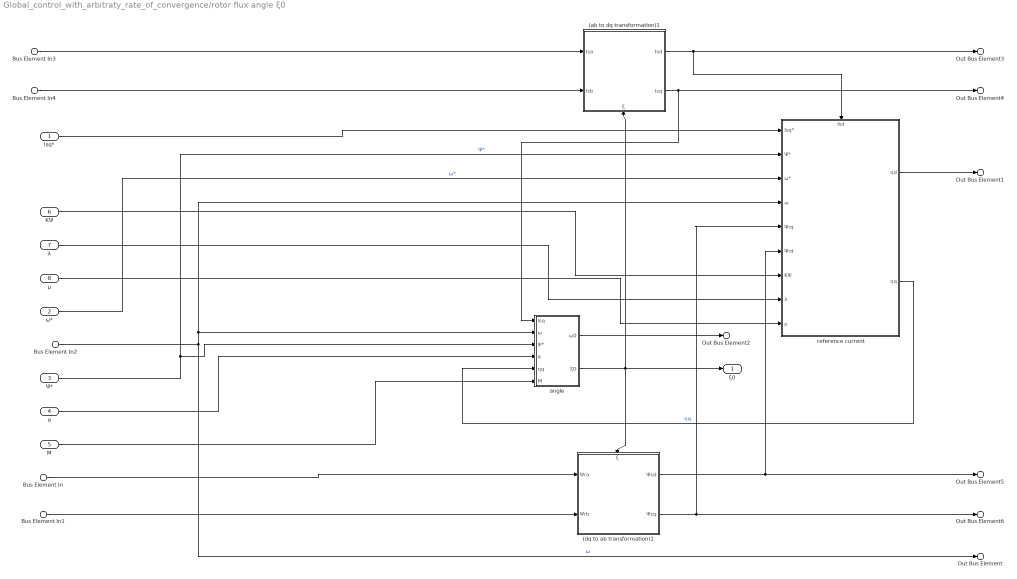
== system Global_control_with_arbitraty_rate_of_convergence/rotor flux angle ξ0 ==
  Isq* : Inport
  ω* : Inport  Port=2
  Ψ* : Inport  Port=3
  α : Inport  Port=4
  M : Inport  Port=5
  KΨ : Inport  Port=6
  λ : Inport  Port=7
  µ : Inport  Port=8
  Bus Element In4 : Inport  Port=9  PortName=mesin  Element=Isb
  Bus Element In : Inport  Port=9  PortName=mesin  Element=Ψra
  Bus Element In1 : Inport  Port=9  PortName=mesin  Element=Ψrb
  Bus Element In2 : Inport  Port=9  PortName=mesin  Element=ω
  Bus Element In3 : Inport  Port=9  PortName=mesin  Element=Isa
  (ab to dq transformation)1 : Subsystem
      settings: PortSchema="{\"entries\":[{\"content\":{\"sides\":[{\"content\":{\"connectorIds\":[\"In1\",\"In2\"]},\"type\":\"ConnectorPlacement.EquallySpacedRectSide\",\"uuid\":\"5c330d99-0e0d-44c6-96f8-2a2206da92f9\"},{\"content\":{\"connectorIds\":[\"Out1\",\"Out2\"],\"side\":\"RIGHT\"},\"type\":\"ConnectorPlacement.EquallySpacedRectSide\",\"uuid\":\"d01d6d1d-3c02-43a0-8f85-93fe8d575b38\"},{\"content\":{\"connectorIds\":[],\"side\":\"TOP\"},\"type\":\"ConnectorPlacement.EquallySpacedRectSide\",\"uuid\":\"e1acbeec-a08c-47b9-8afb-d107cbf7174f\"},{\"content\":{\"connectorIds\":[\"In3\"],\"side\":\"BOTTOM\"},\"type\":\"ConnectorPlacement.EquallySpacedRectSide\",\"uuid\":\"e8043408-ca76-4c99-9608-24b05f44ef39\"}]},\"type\":\"ConnectorPlacement.EquallySpacedConnector\",\"uuid\":\"9536c8a8-a5cc-4817-9165-61d2eb9b262d\"}],\"packageUris\":[\"http://schema.mathworks.com/mf0/Connector/R2020b\"],\"version\":\"1.0\"}"
  (dq to ab transformation)1 : Subsystem
      settings: PortSchema="{\"entries\":[{\"content\":{\"sides\":[{\"content\":{\"connectorIds\":[\"In1\",\"In2\"]},\"type\":\"ConnectorPlacement.EquallySpacedRectSide\",\"uuid\":\"5c330d99-0e0d-44c6-96f8-2a2206da92f9\"},{\"content\":{\"connectorIds\":[\"Out1\",\"Out2\"],\"side\":\"RIGHT\"},\"type\":\"ConnectorPlacement.EquallySpacedRectSide\",\"uuid\":\"d01d6d1d-3c02-43a0-8f85-93fe8d575b38\"},{\"content\":{\"connectorIds\":[\"In3\"],\"side\":\"TOP\"},\"type\":\"ConnectorPlacement.EquallySpacedRectSide\",\"uuid\":\"e1acbeec-a08c-47b9-8afb-d107cbf7174f\"},{\"content\":{\"connectorIds\":[],\"side\":\"BOTTOM\"},\"type\":\"ConnectorPlacement.EquallySpacedRectSide\",\"uuid\":\"e8043408-ca76-4c99-9608-24b05f44ef39\"}]},\"type\":\"ConnectorPlacement.EquallySpacedConnector\",\"uuid\":\"9536c8a8-a5cc-4817-9165-61d2eb9b262d\"}],\"packageUris\":[\"http://schema.mathworks.com/mf0/Connector/R2020b\"],\"version\":\"1.0\"}"
  angle : Subsystem
  reference current : Subsystem
      settings: PortSchema="{\"entries\":[{\"content\":{\"sides\":[{\"content\":{\"connectorIds\":[\"In1\",\"In2\",\"In3\",\"In4\",\"In5\",\"In6\",\"In7\",\"In8\",\"In9\"]},\"type\":\"ConnectorPlacement.EquallySpacedRectSide\",\"uuid\":\"20835a9a-3790-4a84-a1cf-3b356ea8ce55\"},{\"content\":{\"connectorIds\":[\"Out1\",\"Out2\"],\"side\":\"RIGHT\"},\"type\":\"ConnectorPlacement.EquallySpacedRectSide\",\"uuid\":\"c7be742b-d8ac-4ccc-8e57-82e64648b197\"},{\"content\":{\"connectorIds\":[\"In10\"],\"side\":\"TOP\"},\"type\":\"ConnectorPlacement.EquallySpacedRectSide\",\"uuid\":\"50541cb9-7339-4b7f-ab09-a0a36464c354\"}]},\"type\":\"ConnectorPlacement.EquallySpacedConnector\",\"uuid\":\"b3e3bb9d-f2d1-405f-a9ca-c5a471d81e39\"}],\"packageUris\":[\"http://schema.mathworks.com/mf0/Connector/R2020b\"],\"version\":\"1.0\"}"
  ξ0 : Outport
  Out Bus Element : Outport  Port=2  PortName=mes  Element=ω
  Out Bus Element1 : Outport  Port=2  PortName=mes  Element=ηd
  Out Bus Element2 : Outport  Port=2  PortName=mes  Element=ω0
  Out Bus Element3 : Outport  Port=2  PortName=mes  Element=Isd
  Out Bus Element4 : Outport  Port=2  PortName=mes  Element=Isq
  Out Bus Element5 : Outport  Port=2  PortName=mes  Element=Ψrd
  Out Bus Element6 : Outport  Port=2  PortName=mes  Element=Ψrq
  wires:
  Ψ*/1 -> angle/3(Ψ*), reference current/2(Ψ*)  "Ψ*"
  Bus Element In2/1 -> Out Bus Element/1, angle/2(ω), reference current/4(ω)  "ω"
  Bus Element In3/1 -> (ab to dq transformation)1/1(Isa)
  Bus Element In4/1 -> (ab to dq transformation)1/2(Isb)
  Bus Element In/1 -> (dq to ab transformation)1/1(Ψra)
  Bus Element In1/1 -> (dq to ab transformation)1/2(Ψrb)
  reference current/2(ηq) -> angle/5(ηq)  "ηq"
  Isq*/1 -> reference current/1(Isq*)
  ω*/1 -> reference current/3(ω*)  "ω*"
  µ/1 -> reference current/9(µ)
  λ/1 -> reference current/8(λ)
  KΨ/1 -> reference current/7(KΨ)
  reference current/1(ηd) -> Out Bus Element1/1
  (ab to dq transformation)1/1(Isd) -> Out Bus Element3/1, reference current/10(Isd)
  (dq to ab transformation)1/1(Ψsd) -> Out Bus Element5/1, reference current/6(Ψrd)
  (dq to ab transformation)1/2(Ψsq) -> Out Bus Element6/1, reference current/5(Ψrq)
  angle/2(ξ0) -> ξ0/1, (dq to ab transformation)1/3(ξ), (ab to dq transformation)1/3(ξ)
  (ab to dq transformation)1/2(Isq) -> angle/1(Isq), Out Bus Element4/1
  α/1 -> angle/4(α)
  M/1 -> angle/6(M)
  angle/1(ω0) -> Out Bus Element2/1

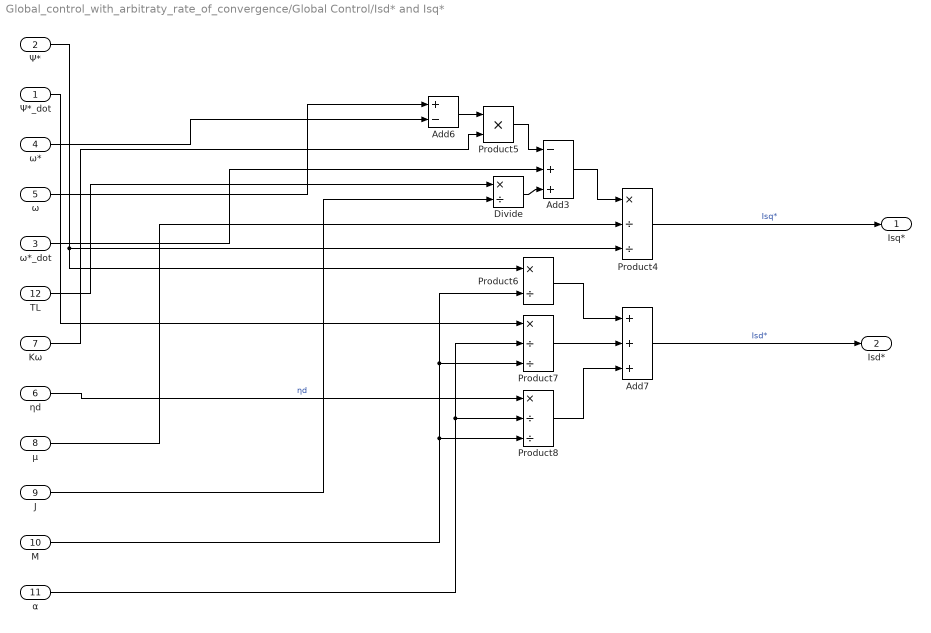
== system Global_control_with_arbitraty_rate_of_convergence/Global Control/Isd* and Isq* ==
  Ψ*_dot : Inport
  Ψ* : Inport  Port=2
  ω*_dot : Inport  Port=3
  ω* : Inport  Port=4
  ω : Inport  Port=5
  ηd : Inport  Port=6
  Kω : Inport  Port=7
  µ : Inport  Port=8
  J : Inport  Port=9
  M : Inport  Port=10
  α : Inport  Port=11
  TL : Inport  Port=12
  Add3 : Sum  Inputs=-++
  Add6 : Sum  Inputs=+-
  Add7 : Sum  Inputs=+++
  Divide : Product  Inputs=*/
  Product4 : Product  Inputs=*//
  Product5 : Product
  Product6 : Product  Inputs=*/
  Product7 : Product  Inputs=*//
  Product8 : Product  Inputs=*//
  Isq* : Outport
  Isd* : Outport  Port=2
  wires:
  Kω/1 -> Product5/2
  M/1 -> Product6/2, Product7/3, Product8/3
  Ψ*/1 -> Product4/3, Product6/1
  µ/1 -> Product4/2
  ηd/1 -> Product8/1  "ηd"
  Divide/1 -> Add3/3
  ω*_dot/1 -> Add3/2
  ω*/1 -> Add6/2
  α/1 -> Product7/2, Product8/2
  Product8/1 -> Add7/3
  J/1 -> Divide/2
  ω/1 -> Add6/1
  Add6/1 -> Product5/1
  Product4/1 -> Isq*/1  "Isq*"
  Add3/1 -> Product4/1
  Ψ*_dot/1 -> Product7/1
  Product5/1 -> Add3/1
  Product6/1 -> Add7/1
  Product7/1 -> Add7/2
  Add7/1 -> Isd*/1  "Isd*"
  TL/1 -> Divide/1

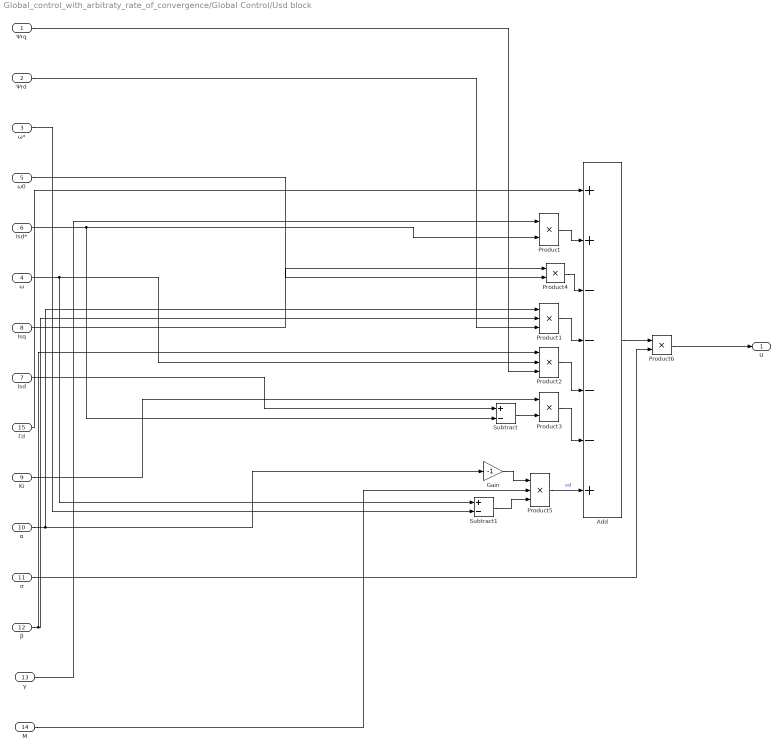
== system Global_control_with_arbitraty_rate_of_convergence/Global Control/Usd block ==
  Ψrq : Inport
  Ψrd : Inport  Port=2
  ω* : Inport  Port=3
  ω : Inport  Port=4
  ω0 : Inport  Port=5
  Isd* : Inport  Port=6
  Isd : Inport  Port=7
  Isq : Inport  Port=8
  Ki : Inport  Port=9
  α : Inport  Port=10
  σ : Inport  Port=11
  β : Inport  Port=12
  γ : Inport  Port=13
  M : Inport  Port=14
  Γd : Inport  Port=15
  Add : Sum  Inputs=++----+
  Gain : Gain  Gain=-1
  Product{,3..4,6} (4 alike) : Product
  Product1 : Product  Inputs=3
  Product2 : Product  Inputs=3
  Product5 : Product  Inputs=3
  Subtract : Sum  Inputs=+-
  Subtract1 : Sum  Inputs=+-
  U : Outport
  wires:
  ω/1 -> Subtract1/1, Product2/2
  Product6/1 -> U/1
  Ψrd/1 -> Product1/3
  Product1/1 -> Add/4
  β/1 -> Product1/2, Product2/1
  Gain/1 -> Product5/1
  Add/1 -> Product6/1
  Product2/1 -> Add/5
  Product3/1 -> Add/6
  Subtract/1 -> Product3/2
  γ/1 -> Product/1
  α/1 -> Product1/1, Gain/1
  M/1 -> Product5/2
  Isd*/1 -> Subtract/2, Product/2
  ω0/1 -> Product4/2
  Product4/1 -> Add/3
  Product5/1 -> Add/7  "vd"
  Product/1 -> Add/2
  Subtract1/1 -> Product5/3
  Ki/1 -> Product3/1
  Isd/1 -> Subtract/1
  σ/1 -> Product6/2
  Ψrq/1 -> Product2/3
  Isq/1 -> Product4/1
  Γd/1 -> Add/1
  ω*/1 -> Subtract1/2

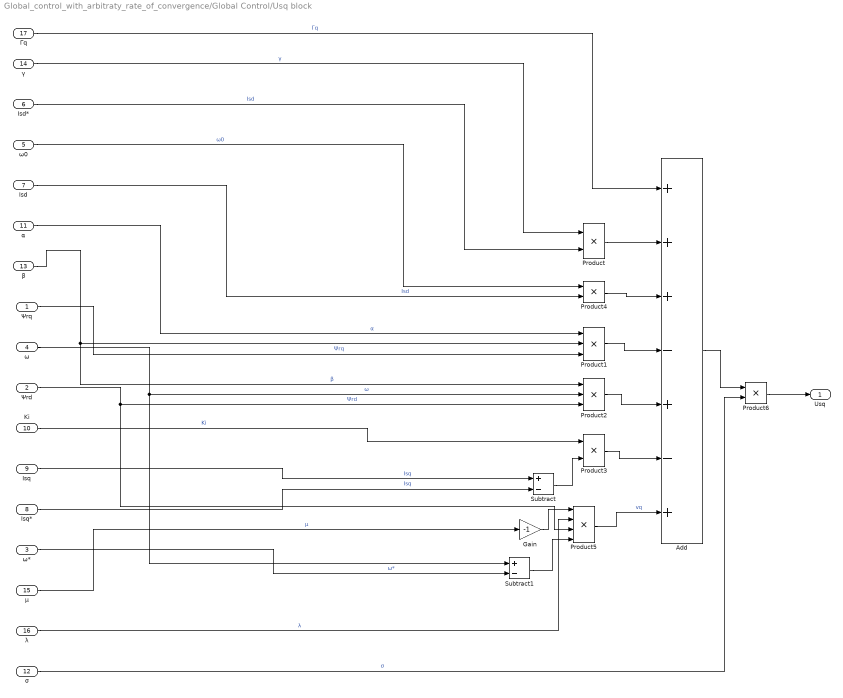
== system Global_control_with_arbitraty_rate_of_convergence/Global Control/Usq block ==
  Ψrq : Inport
  Ψrd : Inport  Port=2
  ω* : Inport  Port=3
  ω : Inport  Port=4
  ω0 : Inport  Port=5
  Isd* : Inport  Port=6
  Isd : Inport  Port=7
  Isq* : Inport  Port=8
  Isq : Inport  Port=9
  Ki : Inport  Port=10
  α : Inport  Port=11
  σ : Inport  Port=12
  β : Inport  Port=13
  γ : Inport  Port=14
  µ : Inport  Port=15
  λ : Inport  Port=16
  Γq : Inport  Port=17
  Add : Sum  Inputs=+++-+-+
  Gain : Gain  Gain=-1
  Product{,3..4,6} (4 alike) : Product
  Product1 : Product  Inputs=3
  Product2 : Product  Inputs=3
  Product5 : Product  Inputs=4
  Subtract : Sum  Inputs=+-
  Subtract1 : Sum  Inputs=+-
  Usq : Outport
  wires:
  Product6/1 -> Usq/1
  Product1/1 -> Add/4
  β/1 -> Product1/2, Product2/1  "β"
  Gain/1 -> Product5/1
  Add/1 -> Product6/1
  Product2/1 -> Add/5
  Product3/1 -> Add/6
  Subtract/1 -> Product3/2
  α/1 -> Product1/1  "α"
  Product4/1 -> Add/3
  Product/1 -> Add/2
  Γq/1 -> Add/1  "Γq"
  γ/1 -> Product/1  "γ"
  Isd*/1 -> Product/2  "Isd"
  ω0/1 -> Product4/1  "ω0"
  Isd/1 -> Product4/2  "Isd"
  Ψrq/1 -> Product1/3  "Ψrq"
  ω/1 -> Subtract1/1, Product2/2  "ω"
  Ψrd/1 -> Product5/3, Product2/3  "Ψrd"
  Ki/1 -> Product3/1  "Ki"
  Isq/1 -> Subtract/1  "Isq"
  Isq*/1 -> Subtract/2  "Isq"
  ω*/1 -> Subtract1/2  "ω*"
  µ/1 -> Gain/1  "µ"
  λ/1 -> Product5/2  "λ"
  Subtract1/1 -> Product5/4
  Product5/1 -> Add/7  "vq"
  σ/1 -> Product6/2  "σ"

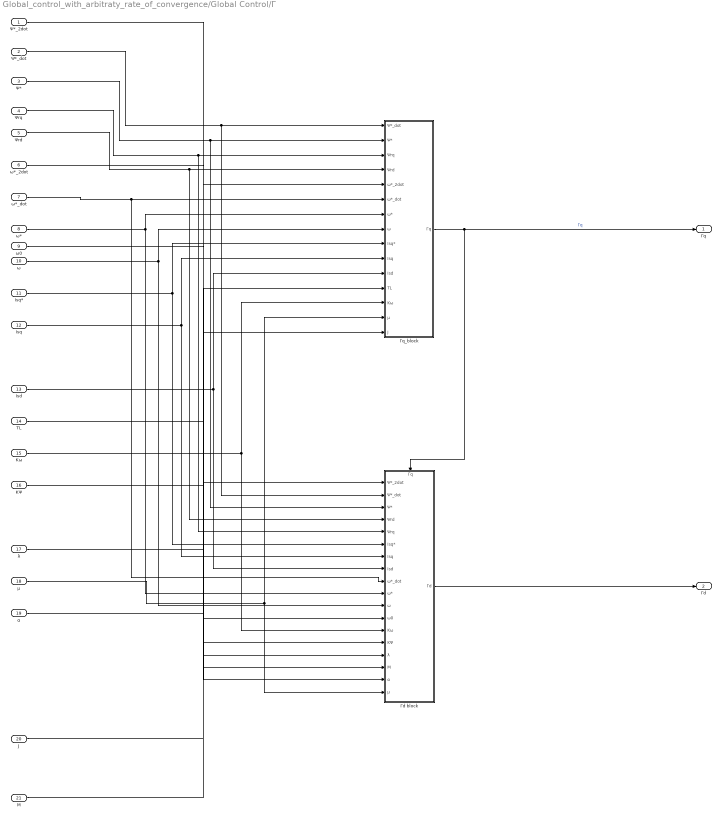
== system Global_control_with_arbitraty_rate_of_convergence/Global Control/Γ ==
  Ψ*_2dot : Inport
  Ψ*_dot : Inport  Port=2
  Ψ* : Inport  Port=3
  Ψrq : Inport  Port=4
  Ψrd : Inport  Port=5
  ω*_2dot : Inport  Port=6
  ω*_dot : Inport  Port=7
  ω* : Inport  Port=8
  ω0 : Inport  Port=9
  ω : Inport  Port=10
  Isq* : Inport  Port=11
  Isq : Inport  Port=12
  Isd : Inport  Port=13
  TL : Inport  Port=14
  Kω : Inport  Port=15
  KΨ : Inport  Port=16
  λ : Inport  Port=17
  µ : Inport  Port=18
  α : Inport  Port=19
  J : Inport  Port=20
  M : Inport  Port=21
  Γd block : Subsystem
      settings: PortSchema="{\"entries\":[{\"content\":{\"sides\":[{\"content\":{\"connectorIds\":[\"In1\",\"In2\",\"In3\",\"In4\",\"In5\",\"In6\",\"In7\",\"In8\",\"In9\",\"In10\",\"In11\",\"In12\",\"In13\",\"In14\",\"In15\",\"In16\",\"In17\",\"In18\"]},\"type\":\"ConnectorPlacement.EquallySpacedRectSide\",\"uuid\":\"6c103e2d-eef5-457d-ab16-617f51de2bb6\"},{\"content\":{\"connectorIds\":[\"Out1\"],\"side\":\"RIGHT\"},\"type\":\"ConnectorPlacement.EquallySpacedRectSide\",\"uuid\":\"d0060888-85cb-49dc-96d4-360cb55f979d\"},{\"content\":{\"connectorIds\":[\"In19\"],\"side\":\"TOP\"},\"type\":\"ConnectorPlacement.EquallySpacedRectSide\",\"uuid\":\"c309ca79-9ccc-4e7a-81b6-dbd7fe2c6fbb\"}]},\"type\":\"ConnectorPlacement.EquallySpacedConnector\",\"uuid\":\"e9330f3c-ebb7-4d09-a354-84c6ad186824\"}],\"packageUris\":[\"http://schema.mathworks.com/mf0/Connector/R2020b\"],\"version\":\"1.0\"}"
  Γq_block : Subsystem
  Γq : Outport
  Γd : Outport  Port=2
  wires:
  Ψ*_dot/1 -> Γd block/2(Ψ*_dot), Γq_block/1(Ψ*_dot)
  Ψrq/1 -> Γd block/5(Ψrq), Γq_block/3(Ψrq)
  Γd block/1(Γd) -> Γd/1
  Ψrd/1 -> Γd block/4(Ψrd), Γq_block/4(Ψrd)
  ω/1 -> Γd block/11(ω), Γq_block/8(ω)
  Γq_block/1(Γq) -> Γq/1, Γd block/19(Γq)  "Γq"
  Isd/1 -> Γd block/8(Isd), Γq_block/11(Isd)
  Isq*/1 -> Γd block/6(Isq*), Γq_block/9(Isq*)
  ω*/1 -> Γd block/10(ω*), Γq_block/7(ω*)
  Kω/1 -> Γd block/13(Kω), Γq_block/13(Kω)
  Isq/1 -> Γd block/7(Isq), Γq_block/10(Isq)
  KΨ/1 -> Γd block/14(KΨ)
  α/1 -> Γd block/17(α)
  λ/1 -> Γd block/15(λ)
  µ/1 -> Γq_block/14(µ), Γd block/18(µ)
  ω*_dot/1 -> Γq_block/6(ω*_dot), Γd block/9(ω*_dot)
  Ψ*/1 -> Γd block/3(Ψ*), Γq_block/2(Ψ*)
  M/1 -> Γd block/16(M)
  Ψ*_2dot/1 -> Γd block/1(Ψ*_2dot)
  J/1 -> Γq_block/15(J)
  ω0/1 -> Γd block/12(ω0)
  ω*_2dot/1 -> Γq_block/5(ω*_2dot)
  TL/1 -> Γq_block/12(TL)

== system Global_control_with_arbitraty_rate_of_convergence/rotor flux angle ξ0/(ab to dq transformation)1 ==
  Isa : Inport
  Isb : Inport  Port=2
  ξ : Inport  Port=3
  Cos : Trigonometry  Operator=cos
  Cos1 : Trigonometry
  Product{,1..3} (4 alike) : Product
  Sin : Trigonometry
  Sin1 : Trigonometry  Operator=cos
  Subtract : Sum
  Subtract1 : Sum  Inputs=-+
  Isd : Outport
  Isq : Outport  Port=2
  wires:
  Subtract1/1 -> Isq/1  "Isb"
  Subtract/1 -> Isd/1  "Isa"
  ξ/1 -> Sin1/1, Cos1/1, Sin/1, Cos/1  "ξ"
  Cos/1 -> Product/1
  Sin/1 -> Product1/2
  Cos1/1 -> Product2/1
  Sin1/1 -> Product3/2
  Isa/1 -> Product2/2, Product/2
  Isb/1 -> Product3/1, Product1/1
  Product/1 -> Subtract/1
  Product1/1 -> Subtract/2
  Product2/1 -> Subtract1/1
  Product3/1 -> Subtract1/2

== system Global_control_with_arbitraty_rate_of_convergence/rotor flux angle ξ0/(dq to ab transformation)1 ==
  Ψra : Inport
  Ψrb : Inport  Port=2
  ξ : Inport  Port=3
  Cos : Trigonometry  Operator=cos
  Cos1 : Trigonometry
  Product{,1..3} (4 alike) : Product
  Sin : Trigonometry
  Sin1 : Trigonometry  Operator=cos
  Subtract : Sum
  Subtract1 : Sum  Inputs=-+
  Ψsd : Outport
  Ψsq : Outport  Port=2
  wires:
  Subtract1/1 -> Ψsq/1
  Subtract/1 -> Ψsd/1
  ξ/1 -> Sin1/1, Cos1/1, Sin/1, Cos/1  "ξ"
  Cos/1 -> Product/1
  Sin/1 -> Product1/2
  Cos1/1 -> Product2/1
  Sin1/1 -> Product3/2
  Ψra/1 -> Product2/2, Product/2
  Ψrb/1 -> Product3/1, Product1/1
  Product/1 -> Subtract/1
  Product1/1 -> Subtract/2
  Product2/1 -> Subtract1/1
  Product3/1 -> Subtract1/2

== system Global_control_with_arbitraty_rate_of_convergence/rotor flux angle ξ0/angle ==
  Isq : Inport
  ω : Inport  Port=2
  Ψ* : Inport  Port=3
  α : Inport  Port=4
  ηq : Inport  Port=5
  M : Inport  Port=6
  Add : Sum  Inputs=++-
  Discrete-Time Integrator : DiscreteIntegrator  SampleTime=-1  ICPrevOutput=DiscIntNeverNeededParam  ICPrevScaledInput=DiscIntNeverNeededParam
  Product : Product  Inputs=***/
  Product1 : Product  Inputs=*/
  ω0 : Outport
  ξ0 : Outport  Port=2
  wires:
  Ψ*/1 -> Product/4, Product1/2
  M/1 -> Product/3
  ω/1 -> Add/2
  α/1 -> Product/2
  Product/1 -> Add/1
  Discrete-Time Integrator/1 -> ξ0/1
  Add/1 -> ω0/1, Discrete-Time Integrator/1
  Product1/1 -> Add/3
  ηq/1 -> Product1/1
  Isq/1 -> Product/1

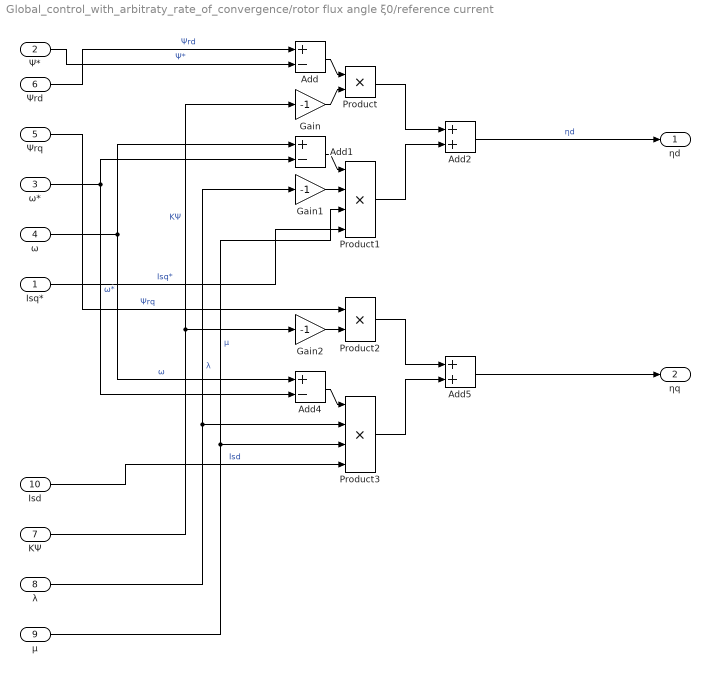
== system Global_control_with_arbitraty_rate_of_convergence/rotor flux angle ξ0/reference current ==
  Isq* : Inport
  Ψ* : Inport  Port=2
  ω* : Inport  Port=3
  ω : Inport  Port=4
  Ψrq : Inport  Port=5
  Ψrd : Inport  Port=6
  KΨ : Inport  Port=7
  λ : Inport  Port=8
  µ : Inport  Port=9
  Isd : Inport  Port=10
  Add : Sum  Inputs=+-
  Add1 : Sum  Inputs=+-
  Add2 : Sum
  Add4 : Sum  Inputs=+-
  Add5 : Sum
  Gain : Gain  Gain=-1
  Gain1 : Gain  Gain=-1
  Gain2 : Gain  Gain=-1
  Product : Product
  Product1 : Product  Inputs=4
  Product2 : Product
  Product3 : Product  Inputs=4
  ηd : Outport
  ηq : Outport  Port=2
  wires:
  Ψrd/1 -> Add/1  "Ψrd"
  Ψ*/1 -> Add/2  "Ψ*"
  Add/1 -> Product/1
  Gain/1 -> Product/2
  KΨ/1 -> Gain2/1, Gain/1  "KΨ"
  Add1/1 -> Product1/1
  Gain1/1 -> Product1/2
  ω/1 -> Add4/1, Add1/1  "ω"
  ω*/1 -> Add4/2, Add1/2  "ω*"
  λ/1 -> Gain1/1, Product3/2  "λ"
  µ/1 -> Product3/3, Product1/3  "µ"
  Product/1 -> Add2/1
  Product1/1 -> Add2/2
  Add2/1 -> ηd/1  "ηd"
  Add4/1 -> Product3/1
  Product3/1 -> Add5/2
  Product2/1 -> Add5/1
  Gain2/1 -> Product2/2
  Ψrq/1 -> Product2/1  "Ψrq"
  Isd/1 -> Product3/4  "Isd"
  Add5/1 -> ηq/1
  Isq*/1 -> Product1/4  "Isq*"

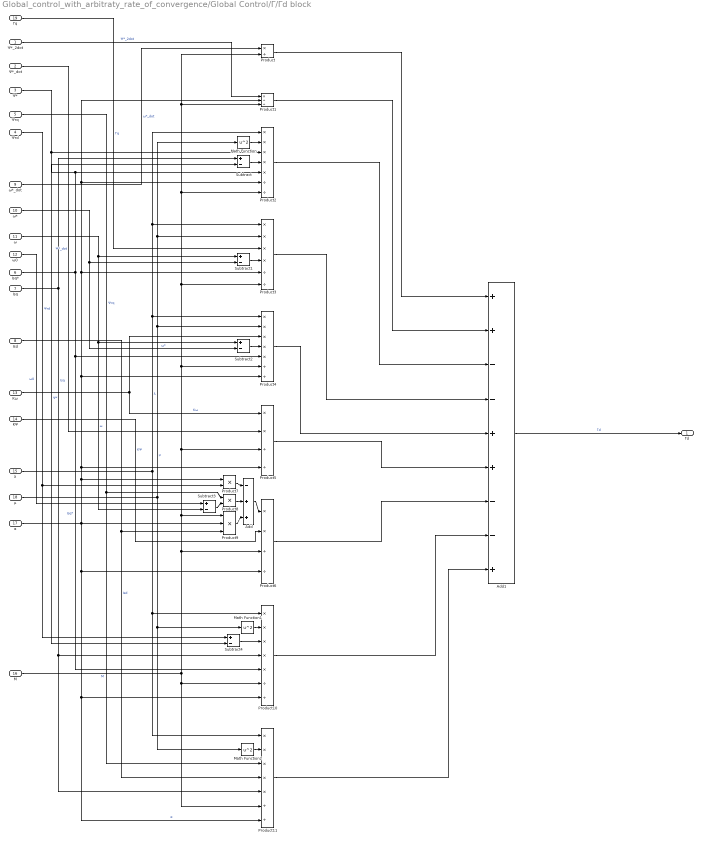
== system Global_control_with_arbitraty_rate_of_convergence/Global Control/Γ/Γd block ==
  Ψ*_2dot : Inport
  Ψ*_dot : Inport  Port=2
  Ψ* : Inport  Port=3
  Ψrd : Inport  Port=4
  Ψrq : Inport  Port=5
  Isq* : Inport  Port=6
  Isq : Inport  Port=7
  Isd : Inport  Port=8
  ω*_dot : Inport  Port=9
  ω* : Inport  Port=10
  ω : Inport  Port=11
  ω0 : Inport  Port=12
  Kω : Inport  Port=13
  KΨ : Inport  Port=14
  λ : Inport  Port=15
  M : Inport  Port=16
  α : Inport  Port=17
  µ : Inport  Port=18
  Γq : Inport  Port=19
  Add : Sum  Inputs=-++
  Add1 : Sum  Inputs=++--++--+
  Math Function : Math  Operator=square  SaturateOnIntegerOverflow=on
  Math Function1 : Math  Operator=square  SaturateOnIntegerOverflow=on
  Math Function2 : Math  Operator=square  SaturateOnIntegerOverflow=on
  Product : Product  Inputs=*/
  Product1 : Product  Inputs=*//
  Product{2,4,10..11} (4 alike) : Product  Inputs=*****//
  Product3 : Product  Inputs=****//
  Product5 : Product  Inputs=**//
  Product6 : Product  Inputs=**//
  Product7 : Product
  Product8 : Product
  Product9 : Product  Inputs=3
  Subtract{,1..4} (5 alike) : Sum  Inputs=+-
  Γd : Outport
  wires:
  ω*_dot/1 -> Product/1  "ω*_dot"
  M/1 -> Product11/6, Product10/6, Product9/1, Product5/3, Product4/6, Product3/6, Product2/7, Product1/3, Product/2, Product6/3  "M"
  Ψ*_2dot/1 -> Product1/1  "Ψ*_2dot"
  α/1 -> Product11/7, Product10/7, Product6/4, Product9/2, Product7/1, Product4/7, Product1/2, Product2/6, Product3/5, Product5/4  "α"
  λ/1 -> Product11/1, Product10/1, Product4/1, Product3/1, Product2/1  "λ"
  Math Function/1 -> Product2/2
  µ/1 -> Math Function2/1, Math Function1/1, Math Function/1, Product3/2, Product4/2  "µ"
  Ψ*/1 -> Product2/3, Subtract4/2  "Ψ*"
  Subtract/1 -> Product2/4
  Isq*/1 -> Subtract/2, Product2/5, Product10/5, Product4/5  "Isq*"
  Isq/1 -> Product11/5, Product10/4, Subtract/1  "Isq"
  Γq/1 -> Product3/3  "Γq"
  Subtract1/1 -> Product3/4
  ω/1 -> Subtract3/2, Subtract2/1, Subtract1/1  "ω"
  ω*/1 -> Subtract2/2, Subtract1/2  "ω*"
  Subtract2/1 -> Product4/4
  Kω/1 -> Product5/1, Product4/3  "Kω"
  Ψ*_dot/1 -> Product5/2  "Ψ*_dot"
  KΨ/1 -> Product6/2  "KΨ"
  Add/1 -> Product6/1
  Product7/1 -> Add/1
  Ψrd/1 -> Subtract4/1, Product7/2  "Ψrd"
  Product8/1 -> Add/2
  Subtract3/1 -> Product8/2
  Ψrq/1 -> Product11/3, Product8/1  "Ψrq"
  ω0/1 -> Subtract3/1  "ω0"
  Product9/1 -> Add/3
  Isd/1 -> Product11/4, Product9/3  "Isd"
  Math Function1/1 -> Product10/2
  Subtract4/1 -> Product10/3
  Math Function2/1 -> Product11/2
  Product/1 -> Add1/1
  Product1/1 -> Add1/2
  Product2/1 -> Add1/3
  Add1/1 -> Γd/1  "Γd"
  Product3/1 -> Add1/4
  Product4/1 -> Add1/5
  Product5/1 -> Add1/6
  Product6/1 -> Add1/7
  Product10/1 -> Add1/8
  Product11/1 -> Add1/9
